simulink model "Vorlage_Gesamtanlage_v27"  (R2021a)
settings: Solver=ode3  StartTime=0.0  StopTime=400  FixedStep=0.01  MaxStep=1  MinStep=0.005  RelTol=1e-3  AbsTol=10  EnableMultiTasking=on
undefined symbols (not defined in the file): A, Flaschengroesse, I, igetr, K, Limits, MaxFlaschen, MRK, numA, PassSilo1, PassSilo2, PHI, Ra, SizeSilo1, SizeSilo2, U, v_band_abfuhr_set, v_band_arbeit_set, v_band_zufuhr_set, v_umsetzer_greifer_set, v_umsetzer_set, v_ve1_set, v_ve2_set
libraries: simulink x94
(part 3 of 3)

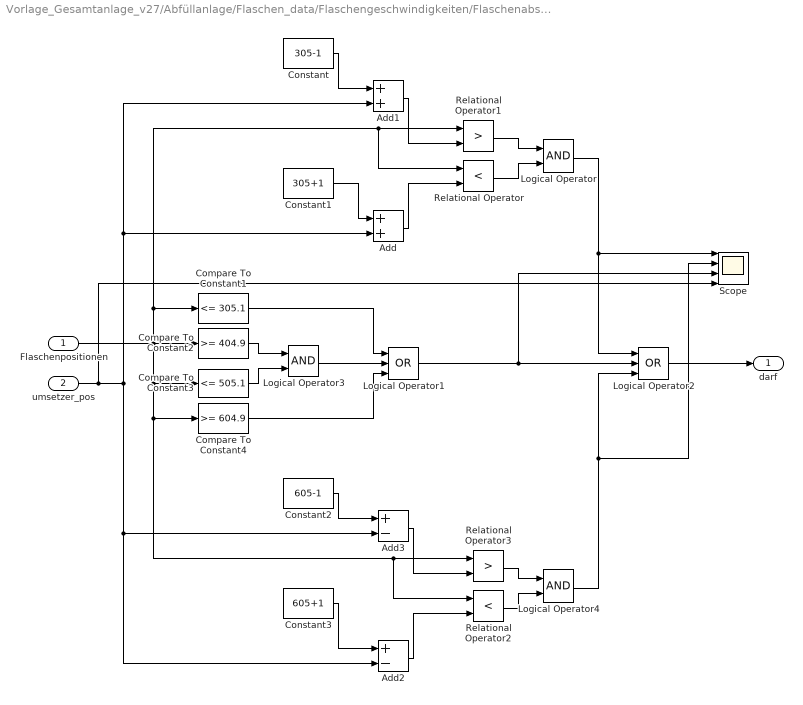
== system Vorlage_Gesamtanlage_v27/Abfüllanlage/Flaschen_data/Flaschengeschwindigkeiten/Flaschenabstandsüberwachung/Umsetzer darf mitnehmen ==
  Flaschenpositionen : Inport
  umsetzer_pos : Inport  Port=2
  Add : Sum
  Add1 : Sum
  Add2 : Sum  Inputs=+-
  Add3 : Sum  Inputs=+-
  Compare To Constant1 : simulink/Logic and Bit Operations/Compare To Constant  relop=<=  const=305.1  OutDataTypeStr=uint8  ZeroCross=off
  Compare To Constant2 : simulink/Logic and Bit Operations/Compare To Constant  relop=>=  const=404.9  OutDataTypeStr=uint8  ZeroCross=off
  Compare To Constant3 : simulink/Logic and Bit Operations/Compare To Constant  relop=<=  const=505.1  OutDataTypeStr=uint8  ZeroCross=off
  Compare To Constant4 : simulink/Logic and Bit Operations/Compare To Constant  relop=>=  const=604.9  OutDataTypeStr=uint8  ZeroCross=off
  Constant : Constant  Value=305-1
  Constant1 : Constant  Value=305+1
  Constant2 : Constant  Value=605-1
  Constant3 : Constant  Value=605+1
  Logical Operator : Logic  AllPortsSameDT=off  OutDataTypeStr=boolean
  Logical Operator1 : Logic  Operator=OR  Inputs=3  AllPortsSameDT=off  OutDataTypeStr=boolean
  Logical Operator2 : Logic  Operator=OR  Inputs=3  AllPortsSameDT=off  OutDataTypeStr=boolean
  Logical Operator3 : Logic  AllPortsSameDT=off  OutDataTypeStr=boolean
  Logical Operator4 : Logic  AllPortsSameDT=off  OutDataTypeStr=boolean
  Relational Operator : RelationalOperator  Operator=<  OutDataTypeStr=boolean  RndMeth=Nearest
  Relational Operator1 : RelationalOperator  Operator=>  OutDataTypeStr=boolean  RndMeth=Nearest
  Relational Operator2 : RelationalOperator  Operator=<  OutDataTypeStr=boolean  RndMeth=Nearest
  Relational Operator3 : RelationalOperator  Operator=>  OutDataTypeStr=boolean  RndMeth=Nearest
  Scope : Scope  NumInputPorts=4
  darf : Outport
  wires:
  Logical Operator2/1 -> darf/1
  Logical Operator1/1 -> Logical Operator2/2, Scope/3
  Compare To Constant1/1 -> Logical Operator1/1
  Logical Operator/1 -> Logical Operator2/1, Scope/1
  Constant/1 -> Add1/1
  Add1/1 -> Relational Operator1/2
  Relational Operator1/1 -> Logical Operator/1
  Relational Operator/1 -> Logical Operator/2
  Add/1 -> Relational Operator/2
  Constant1/1 -> Add/1
  Compare To Constant2/1 -> Logical Operator3/1
  Compare To Constant3/1 -> Logical Operator3/2
  Logical Operator3/1 -> Logical Operator1/2
  Compare To Constant4/1 -> Logical Operator1/3
  Logical Operator4/1 -> Logical Operator2/3, Scope/2
  Constant2/1 -> Add3/1
  Add3/1 -> Relational Operator3/2
  Relational Operator3/1 -> Logical Operator4/1
  Relational Operator2/1 -> Logical Operator4/2
  Add2/1 -> Relational Operator2/2
  Constant3/1 -> Add2/1
  umsetzer_pos/1 -> Add2/2, Add3/2, Add/2, Add1/2, Scope/4
  Flaschenpositionen/1 -> Compare To Constant2/1, Compare To Constant3/1, Compare To Constant4/1, Relational Operator3/1, Relational Operator2/1, Compare To Constant1/1, Relational Operator1/1, Relational Operator/1

== stateflow chart Vorlage_Gesamtanlage_v27/Abfüllanlage/Drehscheibe/Sensor ==
  state Start
    en: beep = 0;
  state Beep
    en: beep=1;
  (default) -> Start
  Start -> Beep : [ml.mod(winkel, 90) <=2 | ml.mod(winkel, 90) >=88]
  Beep -> Start : [ml.mod(winkel, 90) >2 && ml.mod(winkel, 90) <88]
  data: winkel input double; beep output boolean

== stateflow chart Vorlage_Gesamtanlage_v27/Abfüllanlage/Fehlererkennung/Volle Flasche zum Teller zurück/Chart ==
  state Greife_Flasche_Teller
    entry: error = 0;
  state Oeffne_Greifer_Band
  state Warte_auf_VE2
  state Volle_Flasche_gegriffen
  state Greifer_gestartet
    entry: error = 1;
  state Flasche_weg
  (default) -> Greife_Flasche_Teller
  Flasche_weg -> Greife_Flasche_Teller
  Greife_Flasche_Teller -> Oeffne_Greifer_Band : [I_teller_behaelter_hinten == 1 && i_greifer_zu == 1 && i_umsetz_teller == 1]
  Oeffne_Greifer_Band -> Warte_auf_VE2 : [i_greifer_auf == 1 && i_umsetz_band == 1]
  Volle_Flasche_gegriffen -> Greifer_gestartet [order 1] : [o_umsetz_teller==1]
  Warte_auf_VE2 -> Volle_Flasche_gegriffen [order 2] : [i_greifer_zu == 1]
  Warte_auf_VE2 -> Flasche_weg [order 1] : [i_ve2_herein == 1]
  Volle_Flasche_gegriffen -> Flasche_weg [order 2] : after(5,sec)
  data: I_teller_behaelter_hinten input; i_greifer_zu input; i_umsetz_teller input; i_greifer_auf input; i_umsetz_band input; i_ve2_herein input; error output; o_umsetz_teller input

== stateflow chart Vorlage_Gesamtanlage_v27/Steuerung ==
  state Baender [parallel]
    settings: executionOrder=3
    state start
      en:
      o_band[1]=1;
      o_band[2]=0;
    state LT_erkannt
      en:o_band[2]=1;
    state start2
      en:o_band[2]=0;
    (default) -> start
    start -> LT_erkannt : [i_band==1&&(i_umsetzer[4]*i_umsetzer[1]==0)]
    start2 -> LT_erkannt : [(i_umsetzer[4]*i_umsetzer[1]==0)]
    LT_erkannt -> start2 : [i_umsetzer[4]==1&&i_umsetzer[1]==1]
  state Silos [parallel]
    settings: executionOrder=1
    state abfuellen
      en:
      o_silo[1]=1;
      o_silo[2]=1;
    state begin
    state puffer
    state gefuellt
      en:
      o_silo[1]=0;
      o_silo[2]=0;
    state nur_1
      en:
      o_silo[1]=1;
      o_silo[2]=0;
    state nur_2
      en:
      o_silo[1]=0;
      o_silo[2]=1;
    (default) -> begin
    Silos.puffer -> abfuellen [order 1] : [i_silo[3]==0&&i_silo[4]==0]
    begin -> Silos.puffer : [i_silo[2]==1]
    abfuellen -> gefuellt : [i_silo[1]==0]
    nur_1 -> gefuellt : [i_silo[1]==0]
    gefuellt -> begin : [after(2,sec)]
    Silos.puffer -> nur_1 [order 2] : [i_silo[3]==0&&i_silo[4]==1]
    Silos.puffer -> nur_2 [order 3] : [i_silo[3]==1&&i_silo[4]==0]
    nur_2 -> gefuellt : [i_silo[1]==0]
  state Umsetzer [parallel]
    settings: executionOrder=2
    state bewegen_nach_band1
      en:
      o_umsetzer[1]=1;
      o_umsetzer[2]=0;
    state am_band1
      en:
      o_umsetzer[1]=0;
      o_umsetzer[4]=0;
      o_umsetzer[3]=1;
    state keine_flashen_am_teller
    state Anfang
      en:
      o_umsetzer[1]=0;
      o_umsetzer[2]=0;
      o_umsetzer[4]=0;
      o_umsetzer[3]=1;
    state teller_rotieren
    state warten_auf_gefuellt
    state warte
    state bewegen_nach_band
      en:
      o_umsetzer[1]=1;
      o_umsetzer[2]=0;
    state am_band
      en:
      o_umsetzer[1]=0;
      o_umsetzer[4]=0;
      o_umsetzer[3]=1;
    state aus_teller_nehmen
      en:
      o_umsetzer[4]=1;
      o_umsetzer[3]=0;
    state VE1_begin
    state Ende_VE2
    state Warte_VE2
    state naechste_flasche_kommt
      en:
      o_umsetzer[4]=1;
      o_umsetzer[3]=0;
    state bewegen_nach_teller
      en:
      o_umsetzer[1]=0;
      o_umsetzer[2]=1;
    state last_3
    bewegen_nach_band1 -> am_band1 : [i_umsetzer[1]==1]
    keine_flashen_am_teller -> bewegen_nach_band1
    Umsetzer.warte -> keine_flashen_am_teller [order 1] : [i_teller[2]==0]
    (default) -> Umsetzer.Anfang
    am_band1 -> naechste_flasche_kommt : [i_vereinzeler[6]==1]
    warten_auf_gefuellt -> teller_rotieren : [i_teller[1]==0]
    Umsetzer.Anfang -> warten_auf_gefuellt : [i_umsetzer[3]==1]
    teller_rotieren -> Umsetzer.warte : [i_teller[1]==1]
    bewegen_nach_band -> am_band : [i_umsetzer[1]==1]
    Umsetzer.warte -> aus_teller_nehmen [order 2] : [i_teller[2]==1]
    aus_teller_nehmen -> bewegen_nach_band : [i_umsetzer[4]==1]
    bewegen_nach_teller -> Umsetzer.Anfang : [i_umsetzer[2]==1]
    am_band -> Warte_VE2 : [i_umsetzer[3]==1&&i_vereinzeler[4]==0]
    Warte_VE2 -> Ende_VE2 : [i_vereinzeler[4]==1]
    VE1_begin -> naechste_flasche_kommt : [i_vereinzeler[6]==1]
    Ende_VE2 -> VE1_begin [order 1] : [i_vereinzeler[2]==0]
    naechste_flasche_kommt -> bewegen_nach_teller : [i_umsetzer[4]==1]
    Ende_VE2 -> last_3 [order 2] : [i_vereinzeler[5]==0]
    last_3 -> bewegen_nach_teller
  state Teller [parallel]
    settings: executionOrder=4
    state warten
    state warten1
    state keine
    state rotieren
      en:
      o_teller=1;
    state Anfang
      en:
      o_teller=0;
    state warte
    state Nachriseln
    (default) -> rotieren
    Teller.Anfang -> warten1 : after(1,sec)
    keine -> rotieren
    rotieren -> warten : after(0.5,sec)
    Nachriseln -> rotieren : after(2,sec)
    Teller.warte -> keine [order 1] : [i_silo[2]==0]
    warten1 -> Teller.warte : [i_umsetzer[3]==1&&i_umsetzer[2]==1]
    Teller.warte -> Nachriseln [order 2] : [i_silo[1]==0]
    warten -> Teller.Anfang : [i_teller[1]==1]
  state VE1_2 [parallel]
    settings: executionOrder=5
    state nicht_geschlossen1
      en:o_vereinzeler[1]=1;
    state G_am_band_bereit
    state stopp2
      en:
      o_vereinzeler[2]=0;
      o_vereinzeler[1]=0;
    state VE2_begin
      en:
      o_vereinzeler[2]=1;
    state VE2_Stopp
      en:
      o_vereinzeler[2]=0;
    state warte
    state nicht_geschlossen
      en:o_vereinzeler[1]=1;
    state warte1
      en:
      o_vereinzeler[1]=0;
    state puffer
      en:
      o_vereinzeler[1]=0;
    G_am_band_bereit -> nicht_geschlossen1 [order 1] : [i_vereinzeler[5]==1&&i_vereinzeler[6]==0&&i_teller[2]==0]
    (default) -> stopp2
    stopp2 -> G_am_band_bereit : [i_umsetzer[1]==1&&i_umsetzer[3]==1]
    nicht_geschlossen1 -> VE1_2.puffer : [i_vereinzeler[1]==1]
    G_am_band_bereit -> VE2_begin [order 3] : [i_vereinzeler[6]==1&&i_umsetzer[3]==1&&clock>320]
    G_am_band_bereit -> VE2_begin [order 2] : [i_vereinzeler[6]==1&&clock<320]
    VE2_begin -> VE2_Stopp : [i_vereinzeler[3]==1]
    VE1_2.warte -> nicht_geschlossen : [i_teller[2]==0&&i_umsetzer[3]==1&&i_umsetzer[1]==1]
    VE2_Stopp -> VE1_2.warte [order 2] : [i_vereinzeler[5]==1]
    VE2_Stopp -> stopp2 [order 1] : [i_vereinzeler[5]==0]
    VE1_2.puffer -> stopp2 : [i_vereinzeler[6]==1]
    warte1 -> stopp2 : [i_vereinzeler[6]==1]
    nicht_geschlossen -> warte1 : [i_vereinzeler[1]==1]
  (default) -> ?
  data: i_band input boolean; o_band output double size=2; o_vereinzeler output double size=2; o_silo output double size=2; o_umsetzer output double size=4; o_teller output double; i_vereinzeler input boolean size=6; i_silo input boolean size=4; i_umsetzer input boolean size=4; i_teller input boolean size=2; clock input double; baender local double; drehen local double; silo local double; ums local double; ve1 local double; ve2 local double
